simulink library "DWD_TRY_Radiation_Filter"  (R2018b)
settings: Solver=ode45  StartTime=0.0  StopTime=10.0  RelTol=1e-3  EnableMultiTasking=on
undefined symbols (not defined in the file): Solar_Radiation_beam_normal, Solar_Radiation_diffuse_horizontal, Solar_Radiation_diffuse_surface, Solar_Radiation_direct_surface
libraries: simulink_extras x1
settings Model: Creator=lena.frank  LastModifiedBy=P41573
settings DataIOCC: LimitDataPoints=on  SaveFormat=Array  SignalLoggingSaveFormat=ModelDataLogs
settings OptimizationCC: ExpressionDepthLimit=2147483647  LifeSpan=inf
settings DebuggingCC: UnderspecifiedInitializationDetection=Classic  MergeDetectMultiDrivingBlocksExec=none  SolverPrmCheckMsg=warning  FcnCallInpInsideContextMsg=warning  StateNameClashWarn=warning  SFUnexpectedBacktrackingDiag=warning  SFNoUnconditionalDefaultTransitionDiag=warning  SFExecutionAtInitializationDiag=none
settings HardwareCC: ProdBitPerPointer=32  ProdBitPerSizeT=32  ProdBitPerPtrDiffT=32  ProdLargestAtomicFloat=None  ProdIntDivRoundTo=Undefined  ProdEndianess=Unspecified  ProdWordSize=32  ProdHWDeviceType=32-bit Generic
settings ModelReferenceCC: PropagateSignalLabelsOutOfModel=off
settings SFSimCC: SimUseLocalCustomCode=off
settings RTWCC: RTWUseLocalCustomCode=off
settings CodeAppCC: StateflowObjectComments=on
settings GRTTargetCC: TargetLangStandard=C89/C90 (ANSI)  GeneratePreprocessorConditionals=Disable all  CombineOutputUpdateFcns=off  GRTInterface=on
settings ConfigComp: CovMetricSettings=dw  CovHtmlReporting=on  CovSaveCumulativeToWorkspaceVar=on  CovSaveSingleToWorkspaceVar=on  CovExternalEMLEnable=off

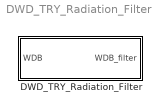
== system DWD_TRY_Radiation_Filter ==
  DWD_TRY_Radiation_Filter : Subsystem  mask(DWD TRY Filter){f=5}
      mask prompts: f "Filter llevel (1 = high, 10 = low)"
      mask help:
      | Filter for solar beam radiation of test reference years 2010 of the german DWD.
      | The original data has some defaults which results in a wrong time-vector (and solar position).
      mask Help: web(fullfile(path_carnot('help'),'DWD_TRY_Radiation_Filter.html'),'-helpbrowser')

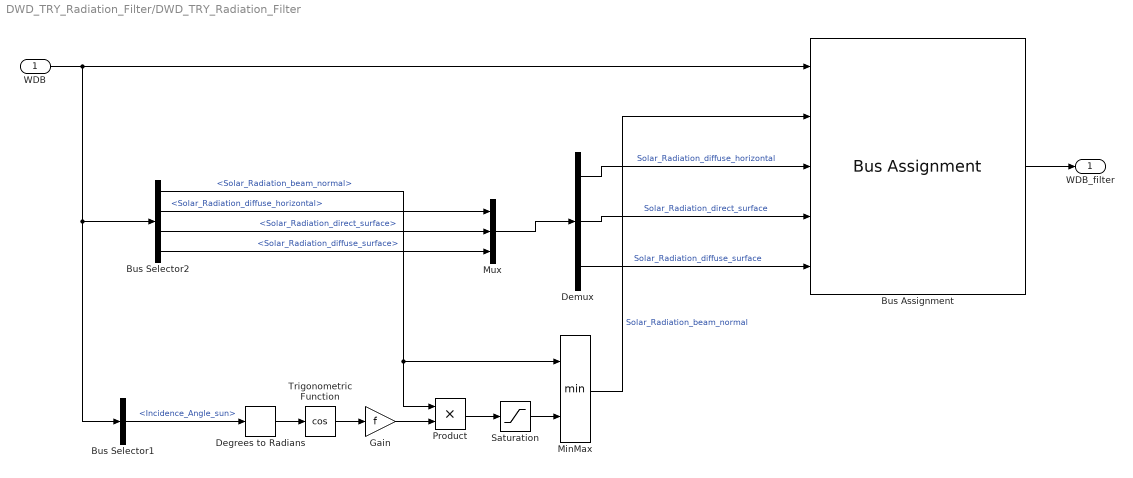
== system DWD_TRY_Radiation_Filter/DWD_TRY_Radiation_Filter ==
  WDB : Inport
  Bus Assignment : BusAssignment  AssignedSignals=Solar_Radiation_beam_normal,Solar_Radiation_diffuse_horizontal,Solar_Radiation_direct_surface,Solar_Radiation_diffuse_surface
  Bus Selector1 : BusSelector  OutputSignals=Incidence_Angle_sun
  Bus Selector2 : BusSelector  OutputSignals=Solar_Radiation_beam_normal,Solar_Radiation_diffuse_horizontal,Solar_Radiation_direct_surface,Solar_Radiation_diffuse_surface
  Degrees to Radians : simulink_extras/Transformations/Degrees to Radians
  Demux : Demux  Outputs=3
  Gain : Gain  Gain=f
  MinMax : MinMax  Inputs=2
  Mux : Mux  Inputs=3
  Product : Product
  Saturation : Saturate  UpperLimit=inf  LowerLimit=0
  Trigonometric Function : Trigonometry  Operator=cos
  WDB_filter : Outport
  wires:
  WDB/1 -> Bus Selector2/1, Bus Selector1/1, Bus Assignment/1
  Bus Assignment/1 -> WDB_filter/1
  Bus Selector1/1 -> Degrees to Radians/1  "<Incidence_Angle_sun>"
  Mux/1 -> Demux/1
  Bus Selector2/3 -> Mux/2  "<Solar_Radiation_direct_surface>"
  Bus Selector2/4 -> Mux/3  "<Solar_Radiation_diffuse_surface>"
  Demux/2 -> Bus Assignment/4  "Solar_Radiation_direct_surface"
  Demux/3 -> Bus Assignment/5  "Solar_Radiation_diffuse_surface"
  Demux/1 -> Bus Assignment/3  "Solar_Radiation_diffuse_horizontal"
  MinMax/1 -> Bus Assignment/2  "Solar_Radiation_beam_normal"
  Bus Selector2/2 -> Mux/1  "<Solar_Radiation_diffuse_horizontal>"
  Bus Selector2/1 -> Product/1, MinMax/1  "<Solar_Radiation_beam_normal>"
  Degrees to Radians/1 -> Trigonometric Function/1
  Trigonometric Function/1 -> Gain/1
  Product/1 -> Saturation/1
  Gain/1 -> Product/2
  Saturation/1 -> MinMax/2
